simulink model "ROBOT_CONTROL_K_POLEPLACE"  (R2023b)
settings: Solver=VariableStepAuto  StartTime=0.0  StopTime=10  RelTol=1e-3
undefined symbols (not defined in the file or in its folder): Alin, Blin, Clin, K, x_init
settings Model: Creator=Kevin  LastModifiedBy=Kevin

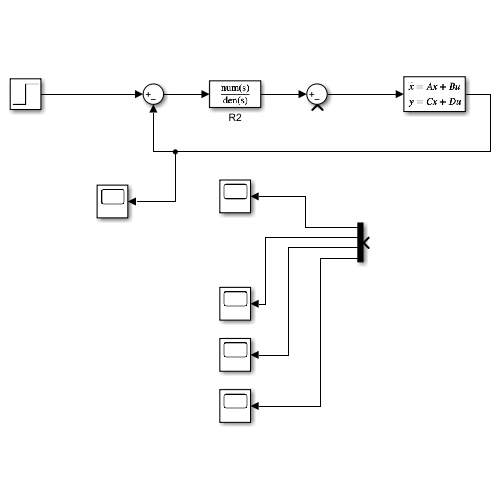
[thumbnail: Simulink's stored preview of the top-level diagram]
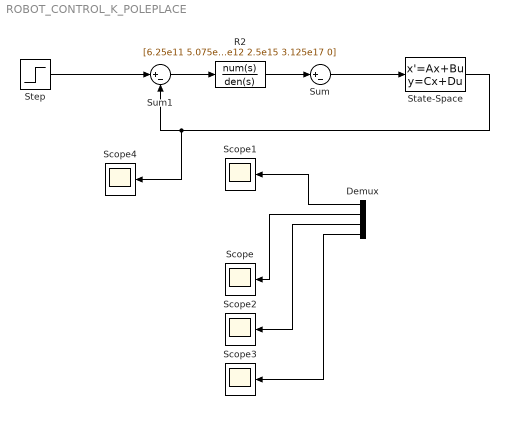
== system ROBOT_CONTROL_K_POLEPLACE ==
  Demux : Demux
  R2 : TransferFcn  Numerator=[6.25e11 5.075e13 1.545e15 2.091e16 1.061e17]  Denominator=[5e06 1e10 7.5e12 2.5e15 3.125e17 0]
  Scope{,1..4} (5 alike) : Scope
  State-Space : StateSpace  A=Alin-Blin*K  B=Blin  C=Clin  D=0  InitialCondition=x_init
  Step : Step  Time=5  After=pi/4  SampleTime=0
  Sum : Sum  Inputs=|+-
  Sum1 : Sum  Inputs=|+-
  wires:
  Sum/1 -> State-Space/1
  Demux/2 -> Scope/1
  Demux/1 -> Scope1/1
  Demux/3 -> Scope2/1
  Demux/4 -> Scope3/1
  State-Space/1 -> Scope4/1, Sum1/2
  Step/1 -> Sum1/1
  Sum1/1 -> R2/1
  R2/1 -> Sum/1
